simulink model "custom_stepper_drive"  (R2013b)
settings: Solver=ode45  StartTime=0.0  StopTime=0.25  FixedStep=Ts  MaxStep=2e-5
PreLoadFcn:
  | assignin('base','Ts',1e-6);
model workspace (MAT data in the model file):
  K_m = 0.4247
  L_0 = 0.00165
  R = 0.77
  D = 0.001
  K_d1 = 0
  K_d2 = 0
  K_d4 = 0
  J = 2.8e-05
  F_s = 0.01
  N_r = 50
  phi_1 = 0
  phi_2 = 0
  start_angle = 0
  start_speed = 0
libraries: simulink x5
Description:
  | Copyright 2008-2013 The MathWorks, Inc.
settings Model: ExtModeAutoUpdateStatusClock=off  Creator=MathWorks  LastModifiedBy=snikitin
settings DataIOCC: SignalLoggingSaveFormat=ModelDataLogs
settings OptimizationCC: ExpressionDepthLimit=2147483647  InitFltsAndDblsToZero=on
settings DebuggingCC: SignalResolutionControl=TryResolveAllWithWarning  FcnCallInpInsideContextMsg=UseLocalSettings  StateNameClashWarn=warning
settings GRTTargetCC: CombineOutputUpdateFcns=off  GRTInterface=on
settings ConfigurationSet: Description=SimMechanics 2G

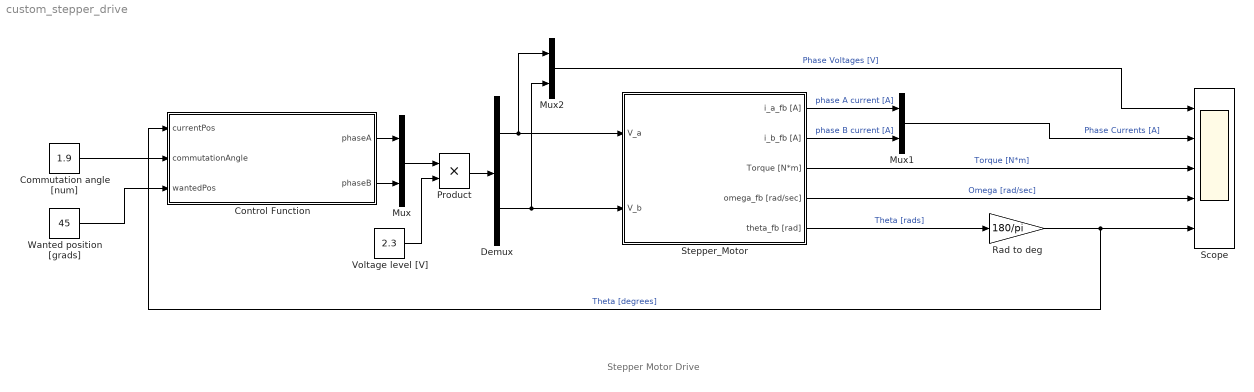
== system custom_stepper_drive ==
  note: Stepper Motor Drive
  Commutation angle [num] : Constant  Value=1.9
  Control Function : MATLAB Function  TreatAsAtomicUnit=on
  Demux : Demux  Outputs=2
  Mux : Mux  Inputs=2
  Mux1 : Mux  Inputs=2
  Mux2 : Mux  Inputs=2
  Product : Product
  Rad to deg : Gain  Gain=180/pi
  Scope : Scope  NumInputPorts=5
      settings: YMin=-5~-5~-5~-5~-5  YMax=5~5~5~5~5
  Stepper_Motor : Subsystem
  Voltage level [V] : Constant  Value=2.3
  Wanted position [grads] : Constant  Value=45
  wires:
  Rad to deg/1 -> Scope/5, Control Function/1(currentPos)  "Theta [degrees]"
  Stepper_Motor/5(theta_fb [rad]) -> Rad to deg/1  "Theta [rads]"
  Control Function/1(phaseA) -> Mux/1
  Control Function/2(phaseB) -> Mux/2
  Wanted position [grads]/1 -> Control Function/3(wantedPos)
  Commutation angle [num]/1 -> Control Function/2(commutationAngle)
  Voltage level [V]/1 -> Product/2
  Mux/1 -> Product/1
  Product/1 -> Demux/1
  Demux/1 -> Mux2/1, Stepper_Motor/1(V_a)
  Demux/2 -> Mux2/2, Stepper_Motor/2(V_b)
  Stepper_Motor/1(i_a_fb [A]) -> Mux1/1  "phase A current [A]"
  Stepper_Motor/2(i_b_fb [A]) -> Mux1/2  "phase B current [A]"
  Stepper_Motor/4(omega_fb [rad/sec]) -> Scope/4  "Omega [rad/sec]"
  Stepper_Motor/3(Torque [N*m]) -> Scope/3  "Torque [N*m]"
  Mux1/1 -> Scope/2  "Phase Currents [A]"
  Mux2/1 -> Scope/1  "Phase Voltages [V]"

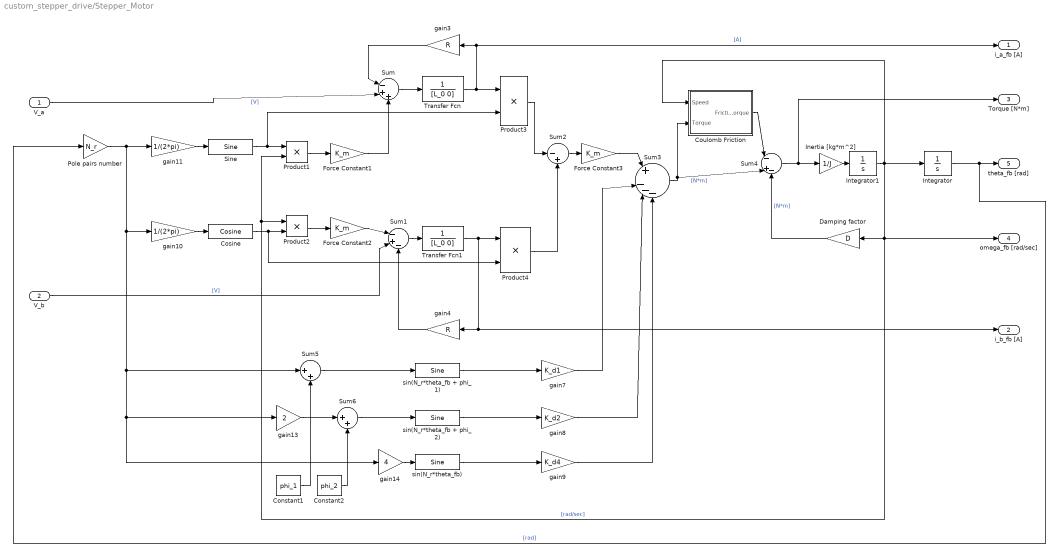
== system custom_stepper_drive/Stepper_Motor ==
  V_a : Inport
  V_b : Inport  Port=2
  Constant1 : Constant  Value=phi_1
  Constant2 : Constant  Value=phi_2
  Cosine : simulink/Lookup Tables/Cosine  Formula=cos(2*pi*u)  NumDataPoints=(2^5)+1  OutputWordLength=16  InternalRulePriority=Speed
  Coulomb Friction : Subsystem
  Damping factor : Gain  Gain=D
  Force Constant1 : Gain  Gain=K_m
  Force Constant2 : Gain  Gain=K_m
  Force Constant3 : Gain  Gain=K_m
  Inertia [kg*m^2] : Gain  Gain=1/J
  Integrator : Integrator  InitialCondition=start_angle
  Integrator1 : Integrator  InitialCondition=start_speed
  Pole pairs number : Gain  Gain=N_r
  Product{1..4} (4 alike) : Product
  Sine : simulink/Lookup Tables/Sine  Formula=sin(2*pi*u)  NumDataPoints=(2^5)+1  OutputWordLength=16  InternalRulePriority=Speed
  Sum : Sum  Inputs=|-++
  Sum1 : Sum  Inputs=|-+-
  Sum2 : Sum  Inputs=|-+
  Sum3 : Sum  Inputs=|+|---
  Sum4 : Sum  Inputs=|-|+-
  Sum5 : Sum  Inputs=|++
  Sum6 : Sum  Inputs=|++
  Transfer Fcn : TransferFcn  Denominator=[L_0 0]
  Transfer Fcn1 : TransferFcn  Denominator=[L_0 0]
  gain10 : Gain  Gain=1/(2*pi)
  gain11 : Gain  Gain=1/(2*pi)
  gain13 : Gain  Gain=2
  gain14 : Gain  Gain=4
  gain3 : Gain  Gain=R
  gain4 : Gain  Gain=R
  gain7 : Gain  Gain=K_d1
  gain8 : Gain  Gain=K_d2
  gain9 : Gain  Gain=K_d4
  sin(N_r*theta_fb + phi_1) : simulink/Lookup Tables/Sine  Formula=sin(2*pi*u)  NumDataPoints=(2^5)+1  OutputWordLength=16  InternalRulePriority=Speed
  sin(N_r*theta_fb + phi_2) : simulink/Lookup Tables/Sine  Formula=sin(2*pi*u)  NumDataPoints=(2^5)+1  OutputWordLength=16  InternalRulePriority=Speed
  sin(N_r*theta_fb) : simulink/Lookup Tables/Sine  Formula=sin(2*pi*u)  NumDataPoints=(2^5)+1  OutputWordLength=16  InternalRulePriority=Speed
  i_a_fb [A] : Outport
  i_b_fb [A] : Outport  Port=2
  Torque [N*m] : Outport  Port=3
  omega_fb [rad/sec] : Outport  Port=4
  theta_fb [rad] : Outport  Port=5
  wires:
  Integrator1/1 -> Product1/2, Product2/1, Damping factor/1, omega_fb [rad/sec]/1, Coulomb Friction/1(Speed), Integrator/1  "[rad/sec]"
  Product1/1 -> Force Constant1/1
  Product2/1 -> Force Constant2/1
  Sum/1 -> Transfer Fcn/1
  Transfer Fcn/1 -> i_a_fb [A]/1, gain3/1, Product3/1  "[A]"
  gain3/1 -> Sum/1
  Force Constant1/1 -> Sum/3
  Sum1/1 -> Transfer Fcn1/1
  Transfer Fcn1/1 -> i_b_fb [A]/1, gain4/1, Product4/1
  gain4/1 -> Sum1/3
  Force Constant2/1 -> Sum1/1
  Product3/1 -> Sum2/1
  Product4/1 -> Sum2/2
  Sum2/1 -> Force Constant3/1
  Sum3/1 -> Sum4/2, Coulomb Friction/2(Torque)  "[N*m]"
  sin(N_r*theta_fb + phi_1)/1 -> gain7/1
  sin(N_r*theta_fb + phi_2)/1 -> gain8/1
  sin(N_r*theta_fb)/1 -> gain9/1
  gain10/1 -> Cosine/1
  gain11/1 -> Sine/1
  Sine/1 -> Product3/2, Product1/1
  Integrator/1 -> Pole pairs number/1, theta_fb [rad]/1  "[rad]"
  Cosine/1 -> Product4/2, Product2/2
  Pole pairs number/1 -> Sum5/1, gain14/1, gain13/1, gain10/1, gain11/1
  gain13/1 -> Sum6/1
  Sum6/1 -> sin(N_r*theta_fb + phi_2)/1
  Sum5/1 -> sin(N_r*theta_fb + phi_1)/1
  gain14/1 -> sin(N_r*theta_fb)/1
  Constant2/1 -> Sum6/2
  Constant1/1 -> Sum5/2
  Force Constant3/1 -> Sum3/1
  gain9/1 -> Sum3/4
  Damping factor/1 -> Sum4/3  "[N*m]"
  Sum4/1 -> Inertia [kg*m^2]/1, Torque [N*m]/1
  gain8/1 -> Sum3/3
  gain7/1 -> Sum3/2
  V_b/1 -> Sum1/2  "[V]"
  V_a/1 -> Sum/2  "[V]"
  Inertia [kg*m^2]/1 -> Integrator1/1
  Coulomb Friction/1(Friction Torque) -> Sum4/1

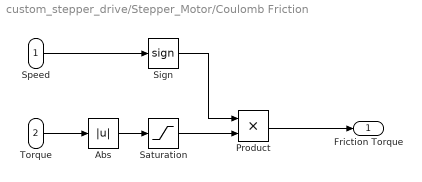
== system custom_stepper_drive/Stepper_Motor/Coulomb Friction ==
  Speed : Inport
  Torque : Inport  Port=2
  Abs : Abs
  Product : Product
  Saturation : Saturate  UpperLimit=F_s  LowerLimit=-F_s
  Sign : Signum
  Friction Torque : Outport
  wires:
  Abs/1 -> Saturation/1
  Saturation/1 -> Product/2
  Sign/1 -> Product/1
  Torque/1 -> Abs/1
  Product/1 -> Friction Torque/1
  Speed/1 -> Sign/1

== matlab function custom_stepper_drive/Control Function ==
  data: currentPos input; commutationAngle input; wantedPos input; phaseA output; phaseB output
function [phaseA, phaseB] = setVoltage(currentPos, commutationAngle, wantedPos)
    persistent initialized;
    persistent lastPhaseA;
    persistent lastPhaseB;
    persistent direction;
    persistent lastActivatedState;
    
    if isempty(initialized)
        lastPhaseA  = 0;
        lastPhaseB  = 0;
        initialized = 1;
        direction   = sign(wantedPos);
        lastActivatedState = nan;
    end

    if (wantedPos - currentPos)*direction <= 0
        phaseA = 0;
        phaseB = 0;
        
        return
    end

    nextPhasesState = calculateNextPhasesState(currentPos, direction, commutationAngle);

    if lastActivatedState ~= nextPhasesState
        [lastPhaseA, lastPhaseB] = setWindingSignals(nextPhasesState);
        lastActivatedState = nextPhasesState;
    end

    phaseA = lastPhaseA;
    phaseB = lastPhaseB;
end

function nextPhasesState = calculateNextPhasesState(currentPosition, direction, commutationAngle) 
    ROTOR_STEP          = 1.8;
    NUMBER_OF_STATES    = 4;
    nextState     = nan;
    
    fuzzyAbsStepNumber          = currentPosition / ROTOR_STEP;
        
    if direction > 0 
        nextState = floor(fuzzyAbsStepNumber + commutationAngle);
    else
        nextState = ceil(fuzzyAbsStepNumber - commutationAngle);
    end
 
    nextPhasesState = mod(nextState, NUMBER_OF_STATES);
end

function [phaseA, phaseB] = setWindingSignals(newState)
    DISABLED            = 0;
    NORMAL_POLARITY     = 1;
    INVERTED_POLARITY   = -1;

    if newState == 0
        phaseA = NORMAL_POLARITY;
        phaseB = DISABLED;

    elseif newState == 1
        phaseA = DISABLED;
        phaseB = NORMAL_POLARITY;

    elseif newState == 2
        phaseA = INVERTED_POLARITY;
        phaseB = DISABLED;

    elseif newState == 3
        phaseA = DISABLED;
        phaseB = INVERTED_POLARITY;

    else
        phaseA = DISABLED;
        phaseB = DISABLED;
        disp('Wrong state recieved')
    end
end
